simulink model "DDSMixer_RTPScalar_Input"  (R2025a)
settings: Solver=VariableStepAuto  StartTime=0.0  StopTime=0.1  RelTol=1e-3
undefined symbols (not defined in the file): aie, dds_mixer, dds_mixer_graph, dsp, mixer, S, vsva2197, xcvc1902, xf
libraries: aieBasic x1, simulink x1, vmcUtilities x1, aieUtilities x1, dspsigops x1
settings Model: Creator=abehbood  LastModifiedBy=sdegala
settings SolverCC: AlgebraicLoopSolver=TrustRegion
settings DebuggingCC: UnconnectedInputMsg=warning  UnconnectedOutputMsg=warning  UnconnectedLineMsg=warning
settings ModelReferenceCC: EnableRefExpFcnMdlSchedulingChecks=on
settings RTWCC: GPUComputeCapability=3.5  DLArmComputeVersion=19.05

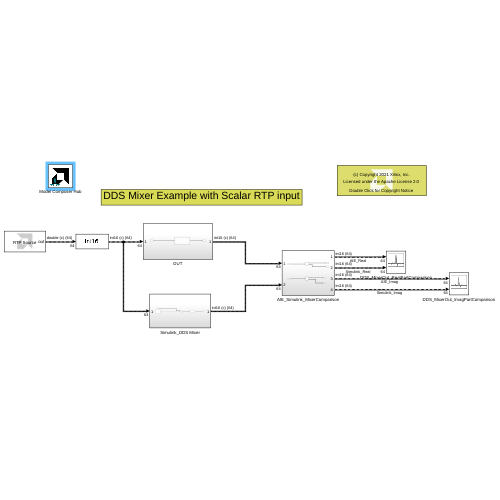
[thumbnail: Simulink's stored preview of the top-level diagram]
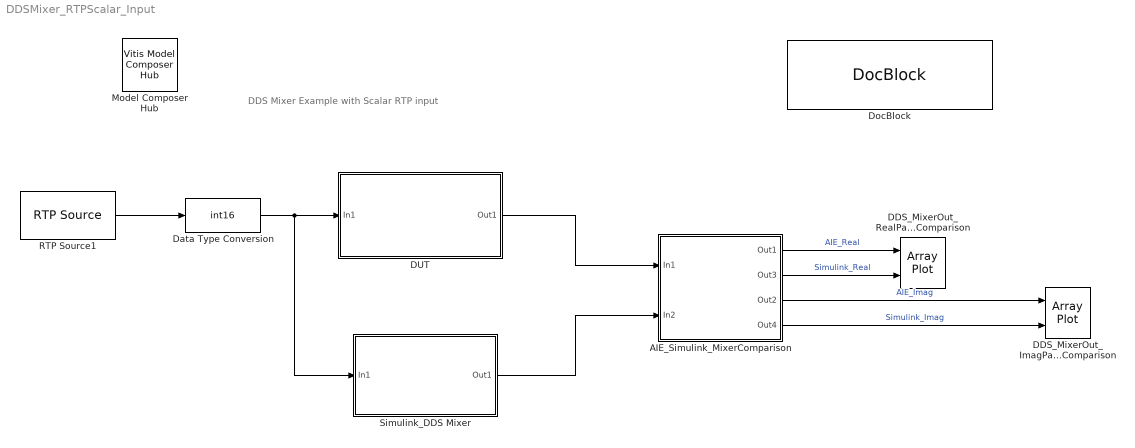
== system DDSMixer_RTPScalar_Input ==
  note: DDS Mixer Example with Scalar RTP input
  AIE_Simulink_MixerComparison : Subsystem
  DDS_MixerOut_ImagPartComparison : ArrayPlot  NumInputPorts=2  WindowPosition=[6.000000,269.000000,845.000000,423.000000,]  ScopeFrameLocation=window  PlotType=Line  YLimits=[-562.5,562.5]  ShowLegend=on
  DDS_MixerOut_RealPartComparison : ArrayPlot  NumInputPorts=2  WindowPosition=[6.000000,41.000000,1272.000000,651.000000,]  ScopeFrameLocation=window  PlotType=Line  YLimits=[-625,625]  ShowLegend=on
  DUT : Subsystem
  Data Type Conversion : DataTypeConversion  OutDataTypeStr=int16  SaturateOnIntegerOverflow=off  RndMeth=Floor
  DocBlock : simulink/Model-Wide Utilities/DocBlock  DocumentType=Text  mask(DocBlock){}
      content=|
      | ///////////////////////////////////////////////////////////////////////////
      | // Copyright 2021 Xilinx
      | //
      | // Licensed under the Apache License, Version 2.0 (the "License");
      | // you may not use this file except in compliance with the License.
      | // You may obtain a copy of the License at
      | //
      | // http://www.apache.org/licenses/LICENSE-2.0
      | //
      | // Unless required by applicable law or agreed to in writing, software
      | // distributed under the License is distributed on an "AS IS" BASIS,
      | // WITHOUT WARRANTIES OR CONDITIONS OF ANY KIND, either express or implied.
      | // See the License for the specific language governing permissions and
      | // limitations under the License.
      | ///////////////////////////////////////////////////////////////////////////
      mask Display:
      | xmcDrawBlockIcon();
      | disp(['{\fontsize{10pt}(c) Copyright 2021' ' Xilinx, Inc.}\newline \newline '],'texmode','on');
      | disp('{\fontsize{10pt}Licensed under the Apache License 2.0}','texmode','on');
      | disp('\newline \newline \newline{\fontsize{10pt}Double Click for Copyright Notice}','texmode','on');
  Model Composer Hub : vmcUtilities/Vitis Model Composer Hub  Tag=genX  CodeGeneration=off  SubsystemName=DUT  BlockHierPath=DDSMixer_RTPScalar_Input/DUT  SubsystemType=AIENode  AIEArrayConfig=Use entire AIE array  StartColumn=1  NumberOfColumns=1  TargetDirectory=./code  exportDesign=on  analyzeDesign=off  validateDesignOnHw=off  ExportType=AI Engines  IpVendor=xilinx.com  IpLibrary=hls  IpVersion=1.0  IpHWLanguage=Verilog  AieCompilerOptions={}  AieSimulatorOptions={}  CreateTestbench=on  TestbenchStackSize=10  RunRtlSim=off  RunCSim=off  RunAieSim=on  AieSimTimeout=50000  RunAieSimProfiling=off  LaunchVitisAnalyzer=off  PlotOutput=off  RunX86Sim=off  X86SimTimeout=10  GenHwImage=off  GenLibadfXo=off  GenHwValidationCode=off  PlatformType=Specify Platform  Platform=/proj/xbuilds/SWIP/9999.0_0818_1732/installs/lin64/2025.2/Vitis/base_platforms/xilinx_vck190_base_202520_1/xilinx_vck190_base_202520_1.xpfm  HwSystemType=Baremetal  HwValidationTarget=hw  ProjDevice=Versal VCK190 Evaluation Platform (xcvc1902-vsva2197-2MP-e-S)  ProjDevicePart=xcvc1902-vsva2197-2MP-e-S  AIEType=AIE  SamplePeriod=-1  ClockFrequency=200  DataPathParallelism=1  xilinxfamily=versalaicore  part=xcvc1902  speed=-2MP-e-S  package=vsva2197  directory=./netlist  testbench=off  incr_netlist=off  synthesis_tool=Vivado  clock_wrapper=Clock Enables  dbl_ovrd=According to Block Masks  dcm_input_clock_period=10  sysclk_period=10  simulink_period=1  eval_field=0  IPInfoJsonString="{\"DUTSubsystemName\":\"DUT\",\"AIESubsystem\":{\"SubsystemName\":\"DUT\",\"TargetDirectory\":\"./code\",\"AIEArrayConfig\":\"Use entire AIE array\",\"StartColumn\":\"0\",\"NumberOfColumns\":\"1\"},\"SubsystemTag\":\"AIENode\"}"  LogFileName=/proj/xhdhdstaff5/sdegala/Head1/HEAD/VMC_2025_2_July/Examples/AIENGINE/Run_Time_Parameters/rtp_scalar/code/model_composer.log  NThreads=4  IPConfigFile=/tmp/vmctmp-6835010160091439353/DDSMixer_RTPScalar_Input_ipconfig.json
  RTP Source1 : aieUtilities/RTP Source  Value=|  SampleTime=1/10e3  OutputForm=Empty
      | [10 + 0i
      | 8 + 5i
      | 3 + 9i
      | -3 + 9i
      | -8 + 5i
      | -10 + 0i
      | -8 - 5i
      | -3 - 9i
      | 3 - 9i
      | 8 - 5i
      | 10 + 0i
      | 8 + 5i
      | 3 + 9i
      | -3 + 9i
      | -8 + 5i
      | -10 + 0i
      | -8 - 5i
      | -3 - 9i
      | 3 - 9i
      | 8 - 5i
      | 10 + 0i
      | 8 + 5i
      | 3 + 9i
      | -3 + 9i
      | -8 + 5i
      | -10 + 0i
      | -8 - 5i
      | -3 - 9i
      | 3 - 9i
      | 8 - 5i
      | 10 + 0i
      | 8 + 5i
      | 3 + 9i
      | -3 + 9i
      | -8 + 5i
      | -10 + 0i
      | -8 - 5i
      | -3 - 9i
      | 3 - 9i
      | 8 - 5i
      | 10 + 0i
      | 8 + 5i
      | 3 + 9i
      | -3 + 9i
      | -8 + 5i
      | -10 + 0i
      | -8 - 5i
      | -3 - 9i
      | 3 - 9i
      | 8 - 5i
      | 10 + 0i
      | 8 + 5i
      | 3 + 9i
      | -3 + 9i
      | -8 + 5i
      | -10 + 0i
      | -8 - 5i
      | -3 - 9i
      | 3 - 9i
      | 8 - 5i
      | 10 + 0i
      | 8 + 5i
      | 3 + 9i
      | -3 + 9i]*50
  Simulink_DDS Mixer : Subsystem
  wires:
  DUT/1(Out1) -> AIE_Simulink_MixerComparison/1(In1)
  AIE_Simulink_MixerComparison/1(Out1) -> DDS_MixerOut_RealPartComparison/1  "AIE_Real"
  AIE_Simulink_MixerComparison/2(Out3) -> DDS_MixerOut_RealPartComparison/2  "Simulink_Real"
  AIE_Simulink_MixerComparison/3(Out2) -> DDS_MixerOut_ImagPartComparison/1  "AIE_Imag"
  AIE_Simulink_MixerComparison/4(Out4) -> DDS_MixerOut_ImagPartComparison/2  "Simulink_Imag"
  RTP Source1/1 -> Data Type Conversion/1
  Data Type Conversion/1 -> Simulink_DDS Mixer/1(In1), DUT/1(In1)
  Simulink_DDS Mixer/1(Out1) -> AIE_Simulink_MixerComparison/2(In2)

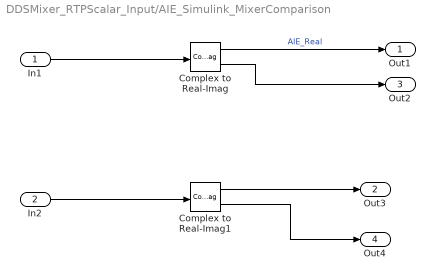
== system DDSMixer_RTPScalar_Input/AIE_Simulink_MixerComparison ==
  In1 : Inport
  In2 : Inport  Port=2
  Complex to Real-Imag : ComplexToRealImag
  Complex to Real-Imag1 : ComplexToRealImag
  Out1 : Outport
  Out3 : Outport  Port=2
  Out2 : Outport  Port=3
  Out4 : Outport  Port=4
  wires:
  In1/1 -> Complex to Real-Imag/1
  Complex to Real-Imag/2 -> Out2/1
  Complex to Real-Imag1/2 -> Out4/1
  Complex to Real-Imag/1 -> Out1/1  "AIE_Real"
  Complex to Real-Imag1/1 -> Out3/1
  In2/1 -> Complex to Real-Imag1/1

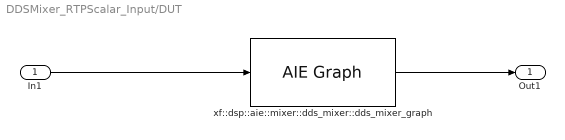
== system DDSMixer_RTPScalar_Input/DUT ==
  In1 : Inport
  xf::dsp::aie::mixer::dds_mixer::dds_mixer_graph : aieBasic/AIE Graph  PortAttributesTable={ 'Input', 'in1[0]', 'stream', 'cint16', '', '', ''; 'Output', 'out[0]', 'stream', 'cint16', '', '', '64' }  PortAttributesEnablement={'off', 'on', 'off', 'off', 'off', 'off', 'off';'off', 'on', 'off', 'off', 'off', 'off', 'on'}  SampleTime=-1  ClassDeclTypeOptions=|  ClassDecl=|  ClassTemplateParams={'TT_DATA', 'typename', 'cint16';'TP_INPUT_WINDOW_VSIZE', 'unsigned int', '64';'TP_MIXER_MODE', 'unsigned int', '1';'TP_API', 'unsigned int', '1';'TP_SSR', 'unsigned int', '1';'TP_RND', 'unsigned int', '4';'TP_SAT', 'unsigned int', '0'}  ClassTemplateParamsEnables={'off', 'off', 'on';'off', 'off', 'on';'off', 'off', 'on';'off', 'off', 'on';'off', 'off', 'on';'off', 'off', 'on';'off', 'off', 'on'}  ClassCtorDeclTypeOptions=C[1 1]@t71@dds_mixer_graph(uint32 const phaseInc, uint32 const initialPhaseOffset)  ClassCtorDecl=dds_mixer_graph(uint32 const phaseInc, uint32 const initialPhaseOffset)  ClassCtorParams={'phaseInc', 'uint32 const', '1000';'initialPhaseOffset', 'uint32 const', '0'}  GraphAllAttrs=|  PortArgDecls={'in stream cint16 in1'; 'out stream cint16 out1'}  PortGraphPortNames={'in1[0]'; 'out[0]'}  HierGraphPortNames={'in1[0]'; 'out[0]'}  PortTypes={'stream'; 'stream'}  PortDataTypes={'cint16'; 'cint16'}  PortSizes={0.000000000000000000e+00; 0.000000000000000000e+00}  PortSynchronicities={'auto'; 'auto'}  PortSignalSizes={0.000000000000000000e+00; 6.400000000000000000e+01}  SimLibPath=''  ClassIndex=1  ClassCtorIndex=1  ClassCtorArgDecls=1000, 0  ClassTabVisible=on  FunctionTabVisible=on  DelayDrawLabels=off  GraphFileSelect=Header file (*.h)  GraphHeaderFile=dds_mixer_graph.hpp  GraphClassName=xf::dsp::aie::mixer::dds_mixer::dds_mixer_graph  GraphName=xf::dsp::aie::mixer::dds_mixer::dds_mixer_graph<cint16, 64, 1, 1, 1, 4, 0>  GraphHeaderFiles={'/proj/xbuilds/SWIP/2023.2_1013_2256/installs/lin64/Model_Composer/2023.2/tps/xf_dsp/L2/include/aie/dds_mixer_graph.hpp'}  GraphSourceFile=./model_composer_work/xmc_aie_lib/d54b6e7b/mygraph.cpp  GraphSearchPaths={'$DSPLIB_ROOT/L1/include/aie', '$DSPLIB_ROOT/L1/src/aie', '$DSPLIB_ROOT/L1/tests/aie/inc/', '$DSPLIB_ROOT/L2/include/aie/'}  GraphPreProcOptions={}  blockJsonConstraints=[]
      ClassDeclTypeOptions=|
      | C[1 1]@t209@template < typename TT_DATA, unsigned int TP_INPUT_WINDOW_VSIZE, unsigned int TP_MIXER_MODE,
      | 				 unsigned int TP_API, unsigned int TP_SSR, unsigned int TP_RND, unsigned int TP_SAT > class dds_mixer_graph
      ClassDecl=|
      | template < typename TT_DATA, unsigned int TP_INPUT_WINDOW_VSIZE, unsigned int TP_MIXER_MODE,
      | 				 unsigned int TP_API, unsigned int TP_SSR, unsigned int TP_RND, unsigned int TP_SAT > class dds_mixer_graph
      GraphAllAttrs=|
      | s[12;12;9;9;19;14;21;23;21;23;24;21;15;17;12;24;26;26;26;27;28;9;21;23;23;23;24;25;14;19;19;29]@FunctionNameDeclFileNamePortNamesPortTypesPortSerializedTypesPortDirectionsPortWindowSizeEnablesPortWindowMarginEnablesPortBufferSizeEnablesPortBufferMarginEnablesPortSynchronicityEnablesPortSignalSizeEnablesPortBufferSizesPortBufferMarginsFunctionDeclFunctionTemplateSpecKindFunctionTemplateParamNamesFunctionTemplateParamKindsFunctionTemplateParamTypesFunctionTemplateParamValuesFunctionTemplateParamEnablesClassDeclClassTemplateSpecKindClassTemplateParamNamesClassTemplateParamKindsClassTemplateParamTypesClassTemplateParamValuesClassTemplateParamEnablesClassCtorDeclsClassCtorParamNamesClassCtorParamTypesClassCtorParamSerializedTypes[1 1]@C[32 1]@nt118@/proj/xbuilds/SWIP/2023.2_1013_2256/installs/lin64/Model_Composer/2023.2/tps/xf_dsp/L2/include/aie/dds_mixer_graph.hppC[3 1]@t3@in1t3@in2t3@outC[3 1]@t80@xf::dsp::aie::mixer::dds_mixer::dds_mixer_graph::portArray< adf::direction::in >t80@xf::dsp::aie::mixer::dds_mixer::dds_mixer_graph::portArray< adf::direction::in >t81@xf::dsp::aie::mixer::dds_mixer::dds_mixer_graph::portArray< adf::direction::out >C[3 1]@t88@{Txf::dsp::aie::mixer::dds_mixer::dds_mixer_graph::portArray{1{t{Sadf::direction::in}}}}t88@{Txf::dsp::aie::mixer::dds_mixer::dds_mixer_graph::portArray{1{t{Sadf::direction::in}}}}t89@{Txf::dsp::aie::mixer::dds_mixer::dds_mixer_graph::portArray{1{t{Sadf::direction::out}}}}C[3 1]@t5@inputt5@inputt5@inputC[3 1]@l0@l0@l0@C[3 1]@l0@l0@l0@C[3 1]@l0@l0@l0@C[3 1]@l0@l0@l0@C[3 1]@l1@l1@l1@C[3 1]@l0@l0@l0@C[3 1]@nnnC[3 1]@nnnt559@namespace xf { namespace dsp { namespace aie { namespace mixer { namespace dds_mixer {
      | template < typename TT_DATA, unsigned int TP_INPUT_WINDOW_VSIZE, unsigned int TP_MIXER_MODE, unsigned int TP_API, unsigned int TP_SSR, unsigned int TP_RND, unsigned int TP_SAT > 
      | void dds_mixer_graph::
      | (xf::dsp::aie::mixer::dds_mixer::dds_mixer_graph::portArray< adf::direction::in > in1, xf::dsp::aie::mixer::dds_mixer::dds_mixer_graph::portArray< adf::direction::in > in2, xf::dsp::aie::mixer::dds_mixer::dds_mixer_graph::portArray< adf::direction::out > out);
      | } } } } }ne[0 1]@e[0 1]@e[0 1]@e[0 1]@e[0 1]@t297@namespace xf { namespace dsp { namespace aie { namespace mixer { namespace dds_mixer {
      | template < typename TT_DATA, unsigned int TP_INPUT_WINDOW_VSIZE, unsigned int TP_MIXER_MODE, unsigned int TP_API, unsigned int TP_SSR, unsigned int TP_RND, unsigned int TP_SAT > class dds_mixer_graph;
      | } } } } }t8@implicitC[7 1]@t7@TT_DATAt21@TP_INPUT_WINDOW_VSIZEt13@TP_MIXER_MODEt6@TP_APIt6@TP_SSRt6@TP_RNDt6@TP_SATC[7 1]@t4@typet7@nontypet7@nontypet7@nontypet7@nontypet7@nontypet7@nontypeC[7 1]@t8@typenamet12@unsigned intt12@unsigned intt12@unsigned intt12@unsigned intt12@unsigned intt12@unsigned intC[7 1]@nnnnnnnC[7 1]@l1@l1@l1@l1@l1@l1@l1@C[1 1]@t71@dds_mixer_graph(uint32 const phaseInc, uint32 const initialPhaseOffset)C[1 1]@C[2 1]@t8@phaseInct18@initialPhaseOffsetC[1 1]@C[2 1]@t12@uint32 constt12@uint32 constC[1 1]@C[2 1]@t10@{Q1{Bu32}}t10@{Q1{Bu32}}
  Out1 : Outport
  wires:
  xf::dsp::aie::mixer::dds_mixer::dds_mixer_graph/1 -> Out1/1
  In1/1 -> xf::dsp::aie::mixer::dds_mixer::dds_mixer_graph/1

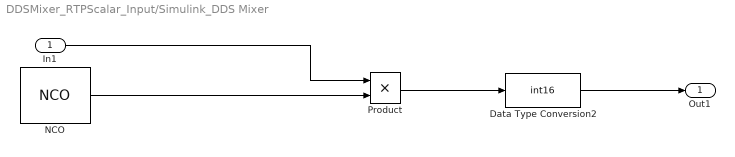
== system DDSMixer_RTPScalar_Input/Simulink_DDS Mixer ==
  In1 : Inport
  Data Type Conversion2 : DataTypeConversion  OutDataTypeStr=int16  SaturateOnIntegerOverflow=off  RndMeth=Floor
  NCO : dspsigops/NCO  AccIncSrc=Specify via dialog  AccInc=1000  PhaseOffsetSrc=Specify via dialog  PhaseOffset=0  AccumWL=32  HasDither=off  DitherWL=4  PNgeneratorLength=19  HasPhaseQuantizer=on  TableDepth=16  HasOutputPhaseError=off  Formula=Complex exponential  DataType=Binary point scaling  OutputWL=16  OutputFL=0  CompMethod=Table lookup (no interpolation)  SampleTime=1  SamplesPerFrame=1  OutputFrames=off
  Product : Product
  Out1 : Outport
  wires:
  NCO/1 -> Product/2
  Product/1 -> Data Type Conversion2/1
  In1/1 -> Product/1
  Data Type Conversion2/1 -> Out1/1
